simulink subsystem "Monitor_Subsystem"  (R2022b)
settings: Solver=VariableStepAuto  StartTime=0.0  StopTime=10.0  RelTol=1e-3
settings Model: Creator=User  LastModifiedBy=Wikian

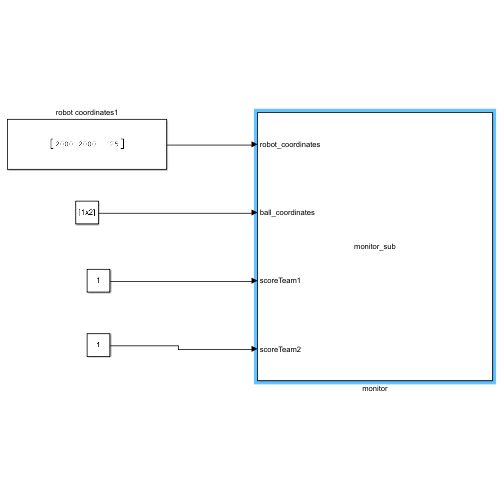
[thumbnail: Simulink's stored preview of the top-level diagram]
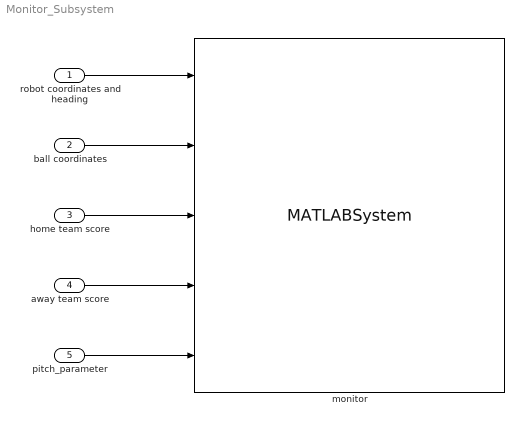
== system Monitor_Subsystem ==
  robot coordinates and heading : Inport
  ball coordinates : Inport  Port=2
  home team score : Inport  Port=3
  away team score : Inport  Port=4
  pitch_parameter : Inport  Port=5
  monitor : MATLABSystem  System=monitor_sub  SimulateUsing=Code generation
      mask Type: monitor_sub
      mask Display:
      | disp('monitor_sub');
      | port_label('input',1,'robot_coordinates');
      | port_label('input',2,'ball_coordinates');
      | port_label('input',3,'scoreTeam1');
      | port_label('input',4,'scoreTeam2');
      | port_label('input',5,'pitchParameters');
  wires:
  robot coordinates and heading/1 -> monitor/1
  home team score/1 -> monitor/3
  ball coordinates/1 -> monitor/2
  away team score/1 -> monitor/4
  pitch_parameter/1 -> monitor/5
